simulink model "LRMate200Experimentor_RobotState"  (R2015b)
settings: Solver=FixedStepDiscrete  StartTime=0.0  StopTime=10.0  FixedStep=si.SolverTimeStep  RelTol=1e-3
model workspace (MATLAB code in the model file):
  | rsi = evalin('base', 'si.ri{1}');
undefined symbols (not defined in the file or in its folder): si
libraries: xpcethercatlib x171
(part 1 of 2)
settings Model: xpc_rtwmakecfg_data=_xpcethercatlib_  ParameterArgumentNames=rsi  Creator=rluser  LastModifiedBy=Chin
settings SolverCC: EnableConcurrentExecution=on
settings DataIOCC: SaveFormat=Array
settings OptimizationCC: BlockReduction=off  OptimizeBlockIOStorage=off  BufferReuse=off  GlobalBufferReuse=off  ExpressionFolding=off  LocalBlockOutputs=off
settings DebuggingCC: SolverPrmCheckMsg=warning
settings HardwareCC: ProdBitPerPointer=32  ProdLargestAtomicFloat=None  ProdWordSize=32  ProdLongLongMode=on  ProdHWDeviceType=Generic->32-bit x86 compatible
settings RTWCC: SystemTargetFile=slrt.tlc  TemplateMakefile=slrt_default_tmf  Description=Simulink Real-Time  RTWCompilerOptimization=on
settings CodeAppCC: MaxIdLength=120
settings SimulinkRealTimeCC: GeneratePreprocessorConditionals=Disable all
settings ConfigComp: CovModelRefEnable=Off  CovSFcnEnable=off

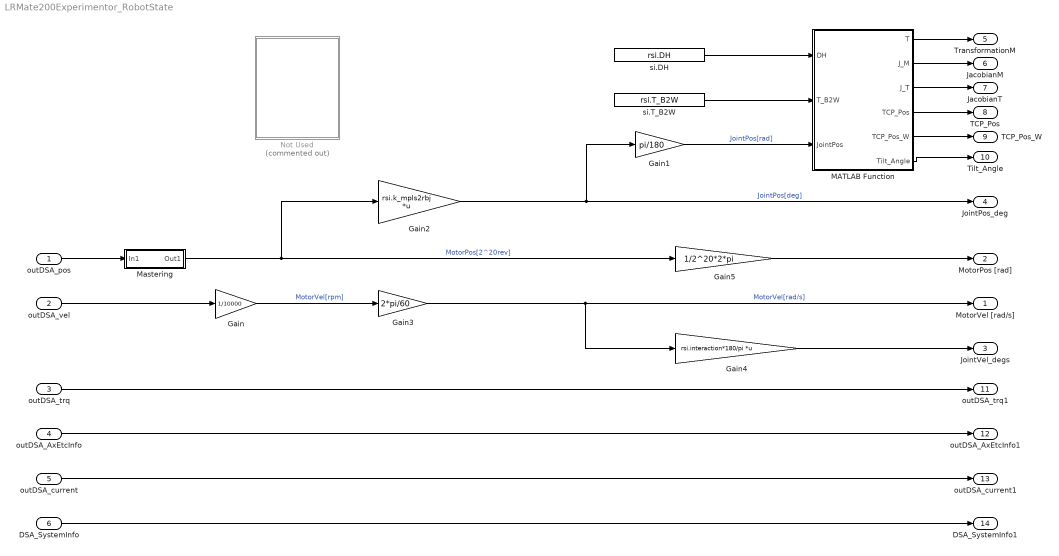
== system LRMate200Experimentor_RobotState ==
  outDSA_pos : Inport  PortDimensions=6
  outDSA_vel : Inport  Port=2  PortDimensions=6
  outDSA_trq : Inport  Port=3  PortDimensions=6
  outDSA_AxEtcInfo : Inport  Port=4  OutDataTypeStr=uint16  PortDimensions=6
  outDSA_current : Inport  Port=5  PortDimensions=6
  DSA_SystemInfo : Inport  Port=6  OutDataTypeStr=uint16
  Gain : Gain  Gain=1/10000  SampleTime=si.tsv
  Gain1 : Gain  Gain=pi/180
  Gain2 : Gain  Gain=rsi.k_mpls2rbj  Multiplication=Matrix(K*u)
  Gain3 : Gain  Gain=2*pi/60
  Gain4 : Gain  Gain=rsi.interaction*180/pi  Multiplication=Matrix(K*u)
  Gain5 : Gain  Gain=1/2^20*2*pi
  MATLAB Function : MATLAB Function  TreatAsAtomicUnit=on
  Mastering : Subsystem
  Not Used : Subsystem  Commented=on
  si.DH : Constant  Value=rsi.DH
  si.T_B2W : Constant  Value=rsi.T_B2W
  MotorVel [rad/s] : Outport
  MotorPos [rad] : Outport  Port=2
  JointVel_degs : Outport  Port=3
  JointPos_deg : Outport  Port=4
  TransformationM : Outport  Port=5
  JacobianM : Outport  Port=6
  JacobianT : Outport  Port=7
  TCP_Pos : Outport  Port=8
  TCP_Pos_W : Outport  Port=9
  Tilt_Angle : Outport  Port=10
  outDSA_trq1 : Outport  Port=11
  outDSA_AxEtcInfo1 : Outport  Port=12
  outDSA_current1 : Outport  Port=13
  DSA_SystemInfo1 : Outport  Port=14
  wires:
  DSA_SystemInfo/1 -> DSA_SystemInfo1/1
  outDSA_current/1 -> outDSA_current1/1
  outDSA_AxEtcInfo/1 -> outDSA_AxEtcInfo1/1
  outDSA_trq/1 -> outDSA_trq1/1
  outDSA_pos/1 -> Mastering/1(In1)
  Gain/1 -> Gain3/1  "MotorVel[rpm]"
  Gain2/1 -> JointPos_deg/1, Gain1/1  "JointPos[deg]"
  Gain3/1 -> MotorVel [rad/s]/1, Gain4/1  "MotorVel[rad/s]"
  si.DH/1 -> MATLAB Function/1(DH)
  MATLAB Function/1(T) -> TransformationM/1
  Gain4/1 -> JointVel_degs/1
  MATLAB Function/2(J_M) -> JacobianM/1
  Gain5/1 -> MotorPos [rad]/1
  Mastering/1(Out1) -> Gain5/1, Gain2/1  "MotorPos[2^20rev]"
  outDSA_vel/1 -> Gain/1
  MATLAB Function/3(J_T) -> JacobianT/1
  Gain1/1 -> MATLAB Function/3(JointPos)  "JointPos[rad]"
  MATLAB Function/4(TCP_Pos) -> TCP_Pos/1
  MATLAB Function/6(Tilt_Angle) -> Tilt_Angle/1
  si.T_B2W/1 -> MATLAB Function/2(T_B2W)
  MATLAB Function/5(TCP_Pos_W) -> TCP_Pos_W/1

== system LRMate200Experimentor_RobotState/Mastering ==
  note: モータ角度
      | [10^6*FlexFeedGear/rev]
  note: モータ角度[2^20/rev]
  note: モータ角度[2^20/rev]
  note: モータ角度[2^19/rev]
  In1 : Inport
  Add : Sum  Inputs=+-
  Gain : Gain  Gain=1./si.DSA_FlexFeedGear/1e6*2^20
  Gain1 : Gain  Gain=2
  MasterCount : Constant  Value=rsi.MasterCount  SampleTime=si.tsv
  Out1 : Outport
  wires:
  MasterCount/1 -> Gain1/1
  In1/1 -> Gain/1
  Add/1 -> Out1/1
  Gain/1 -> Add/1
  Gain1/1 -> Add/2

== system LRMate200Experimentor_RobotState/Not Used ==
  DSA SYSTEM : Subsystem  Commented=on
      settings: MinAlgLoopOccurrences=on
  DSA System Variant : Subsystem  Commented=on  Variant=on
  MATLAB Function : MATLAB Function  TreatAsAtomicUnit=on
  MATLAB Function1 : MATLAB Function  Commented=on  TreatAsAtomicUnit=on

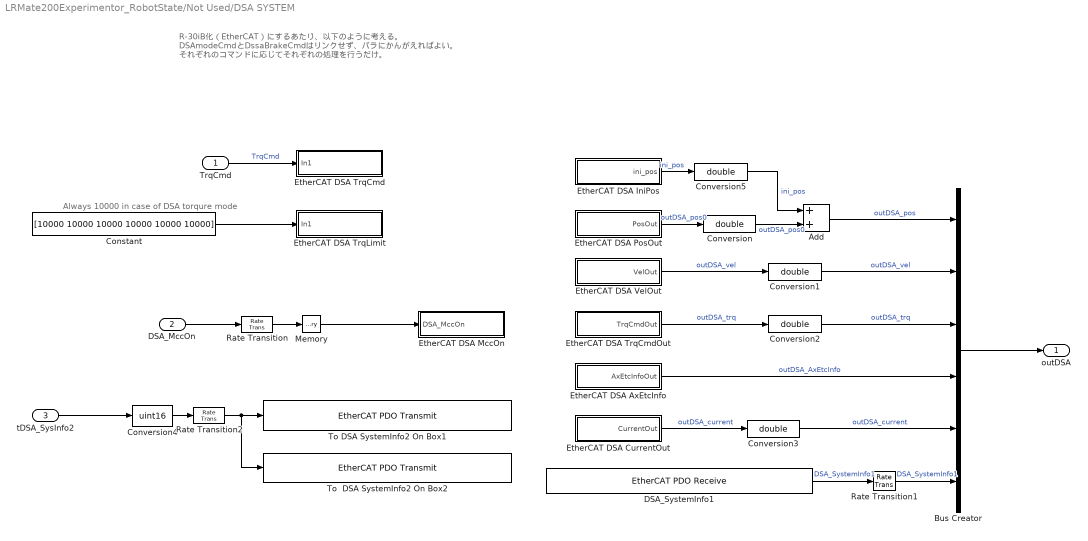
== system LRMate200Experimentor_RobotState/Not Used/DSA SYSTEM ==
  note: Always 10000 in case of DSA torqure mode
  note: R-30iB化（EtherCAT）にするあたり、以下のように考える。
      |
      | DSAmodeCmdとDssaBrakeCmdはリンクせず、パラにかんがえればよい。
      | それぞれのコマンドに応じてそれぞれの処理を行うだけ。
  TrqCmd : Inport
  DSA_MccOn : Inport  Port=2
  tDSA_SysInfo2 : Inport  Port=3
  Add : Sum
  Bus Creator : BusCreator  Inputs=6
  Constant : Constant  Value=[10000 10000 10000 10000 10000 10000]  SampleTime=si.etsv
  Conversion{,1..3,5} (5 alike) : DataTypeConversion  OutDataTypeStr=double
  Conversion4 : DataTypeConversion  OutDataTypeStr=uint16
  DSA_SystemInfo1 : xpcethercatlib/EtherCAT PDO Receive  Priority=2  sig_name=Box 1 (Degital Servo Adapter).NS-IN-SYS-DCIF.NSIS01  sig_offset=1352  sig_type=uint16  type_size=16  sig_dim=1  device_id=0  sample_time=0.000250
  EtherCAT DSA AxEtcInfo : Subsystem
  EtherCAT DSA CurrentOut : Subsystem
  EtherCAT DSA IniPos : Subsystem
  EtherCAT DSA MccOn : Subsystem
  EtherCAT DSA PosOut : Subsystem
  EtherCAT DSA TrqCmd : Subsystem
  EtherCAT DSA TrqCmdOut : Subsystem
  EtherCAT DSA TrqLimit : Subsystem
  EtherCAT DSA VelOut : Subsystem
  Memory : Memory
  Rate Transition : RateTransition
  Rate Transition1 : RateTransition  OutPortSampleTime=si.tsv
  Rate Transition2 : RateTransition
  To  DSA SystemInfo2 On Box2 : xpcethercatlib/EtherCAT PDO Transmit   Priority=3  sig_name=Box 2 (Degital Servo Adapter).NS-OUT-SYS-DCIF.NSOS01  sig_offset=3656  sig_type=uint16  type_size=16  sig_dim=1  device_id=0  sample_time=0.000250
  To DSA SystemInfo2 On Box1 : xpcethercatlib/EtherCAT PDO Transmit   Priority=3  sig_name=Box 1 (Degital Servo Adapter).NS-OUT-SYS-DCIF.NSOS01  sig_offset=1352  sig_type=uint16  type_size=16  sig_dim=1  device_id=0  sample_time=0.000250
  outDSA : Outport
  wires:
  EtherCAT DSA VelOut/1(VelOut) -> Conversion1/1  "outDSA_vel"
  EtherCAT DSA PosOut/1(PosOut) -> Conversion/1  "outDSA_pos0"
  EtherCAT DSA TrqCmdOut/1(TrqCmdOut) -> Conversion2/1  "outDSA_trq"
  EtherCAT DSA AxEtcInfo/1(AxEtcInfoOut) -> Bus Creator/4  "outDSA_AxEtcInfo"
  Bus Creator/1 -> outDSA/1
  TrqCmd/1 -> EtherCAT DSA TrqCmd/1(In1)  "TrqCmd"
  Conversion/1 -> Add/2  "outDSA_pos0"
  Conversion1/1 -> Bus Creator/2  "outDSA_vel"
  Conversion2/1 -> Bus Creator/3  "outDSA_trq"
  Memory/1 -> EtherCAT DSA MccOn/1(DSA_MccOn)
  Rate Transition/1 -> Memory/1
  EtherCAT DSA CurrentOut/1(CurrentOut) -> Conversion3/1  "outDSA_current"
  Conversion3/1 -> Bus Creator/5  "outDSA_current"
  DSA_MccOn/1 -> Rate Transition/1
  Rate Transition2/1 -> To  DSA SystemInfo2 On Box2/1, To DSA SystemInfo2 On Box1/1
  Conversion4/1 -> Rate Transition2/1
  tDSA_SysInfo2/1 -> Conversion4/1
  EtherCAT DSA IniPos/1(ini_pos) -> Conversion5/1  "ini_pos"
  Conversion5/1 -> Add/1  "ini_pos"
  Add/1 -> Bus Creator/1  "outDSA_pos"
  DSA_SystemInfo1/1 -> Rate Transition1/1  "DSA_SystemInfo1"
  Constant/1 -> EtherCAT DSA TrqLimit/1(In1)
  Rate Transition1/1 -> Bus Creator/6  "DSA_SystemInfo1"

== system LRMate200Experimentor_RobotState/Not Used/DSA System Variant ==
  note: 1) Add Subsystem or Model blocks as valid variant choices.
      | 2) You cannot connect blocks at this level. At simulation, connectivity is automatically
      | determined, based on the active variant and port name matching.
  MotorTrqCmd[DSA] : Inport
  DSA_MccOn : Inport  Port=2
  tDSA_SysInfo2 : Inport  Port=3
  DSA System (Robot 1) : Subsystem  VariantControl=robot_no == 1
      settings: MinAlgLoopOccurrences=on
  DSA System (Robot 2) : Subsystem  TreatAsAtomicUnit=on  VariantControl=robot_no == 2
      settings: MinAlgLoopOccurrences=on
  Empty : Subsystem  VariantControl=robot_no == 0
  outDSA : Outport

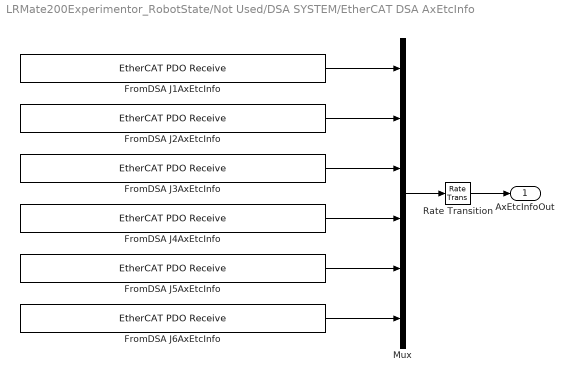
== system LRMate200Experimentor_RobotState/Not Used/DSA SYSTEM/EtherCAT DSA AxEtcInfo ==
  FromDSA J1AxEtcInfo : xpcethercatlib/EtherCAT PDO Receive  Priority=2  sig_name=Box 1 (Degital Servo Adapter).NS-IN-AX01.AX01-NSI07  sig_offset=1704  sig_type=uint16  type_size=16  sig_dim=1  device_id=0  sample_time=0.000250
  FromDSA J2AxEtcInfo : xpcethercatlib/EtherCAT PDO Receive  Priority=2  sig_name=Box 1 (Degital Servo Adapter).NS-IN-AX02.AX02-NSI07  sig_offset=1896  sig_type=uint16  type_size=16  sig_dim=1  device_id=0  sample_time=0.000250
  FromDSA J3AxEtcInfo : xpcethercatlib/EtherCAT PDO Receive  Priority=2  sig_name=Box 1 (Degital Servo Adapter).NS-IN-AX03.AX03-NSI07  sig_offset=2088  sig_type=uint16  type_size=16  sig_dim=1  device_id=0  sample_time=0.000250
  FromDSA J4AxEtcInfo : xpcethercatlib/EtherCAT PDO Receive  Priority=2  sig_name=Box 1 (Degital Servo Adapter).NS-IN-AX04.AX04-NSI07  sig_offset=2280  sig_type=uint16  type_size=16  sig_dim=1  device_id=0  sample_time=0.000250
  FromDSA J5AxEtcInfo : xpcethercatlib/EtherCAT PDO Receive  Priority=2  sig_name=Box 2 (Degital Servo Adapter).NS-IN-AX01.AX01-NSI07  sig_offset=4008  sig_type=uint16  type_size=16  sig_dim=1  device_id=0  sample_time=0.000250
  FromDSA J6AxEtcInfo : xpcethercatlib/EtherCAT PDO Receive  Priority=2  sig_name=Box 2 (Degital Servo Adapter).NS-IN-AX02.AX02-NSI07  sig_offset=4200  sig_type=uint16  type_size=16  sig_dim=1  device_id=0  sample_time=0.000250
  Mux : Mux  Inputs=6
  Rate Transition : RateTransition  OutPortSampleTime=si.tsv
  AxEtcInfoOut : Outport
  wires:
  FromDSA J6AxEtcInfo/1 -> Mux/6
  FromDSA J4AxEtcInfo/1 -> Mux/4
  FromDSA J2AxEtcInfo/1 -> Mux/2
  FromDSA J5AxEtcInfo/1 -> Mux/5
  FromDSA J3AxEtcInfo/1 -> Mux/3
  FromDSA J1AxEtcInfo/1 -> Mux/1
  Mux/1 -> Rate Transition/1
  Rate Transition/1 -> AxEtcInfoOut/1

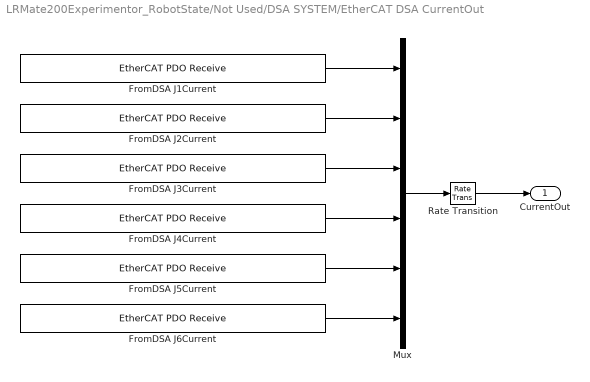
== system LRMate200Experimentor_RobotState/Not Used/DSA SYSTEM/EtherCAT DSA CurrentOut ==
  FromDSA J1Current : xpcethercatlib/EtherCAT PDO Receive  Priority=2  sig_name=Box 1 (Degital Servo Adapter).HS-IN-AX01.AX01-HSI03  sig_offset=360  sig_type=int16  type_size=16  sig_dim=1  device_id=0  sample_time=0.000250
  FromDSA J2Current : xpcethercatlib/EtherCAT PDO Receive  Priority=2  sig_name=Box 1 (Degital Servo Adapter).HS-IN-AX02.AX02-HSI03  sig_offset=616  sig_type=int16  type_size=16  sig_dim=1  device_id=0  sample_time=0.000250
  FromDSA J3Current : xpcethercatlib/EtherCAT PDO Receive  Priority=2  sig_name=Box 1 (Degital Servo Adapter).HS-IN-AX03.AX03-HSI03  sig_offset=872  sig_type=int16  type_size=16  sig_dim=1  device_id=0  sample_time=0.000250
  FromDSA J4Current : xpcethercatlib/EtherCAT PDO Receive  Priority=2  sig_name=Box 1 (Degital Servo Adapter).HS-IN-AX04.AX04-HSI03  sig_offset=1128  sig_type=int16  type_size=16  sig_dim=1  device_id=0  sample_time=0.000250
  FromDSA J5Current : xpcethercatlib/EtherCAT PDO Receive  Priority=2  sig_name=Box 2 (Degital Servo Adapter).HS-IN-AX01.AX01-HSI03  sig_offset=2664  sig_type=int16  type_size=16  sig_dim=1  device_id=0  sample_time=0.000250
  FromDSA J6Current : xpcethercatlib/EtherCAT PDO Receive  Priority=2  sig_name=Box 2 (Degital Servo Adapter).HS-IN-AX02.AX02-HSI03  sig_offset=2920  sig_type=int16  type_size=16  sig_dim=1  device_id=0  sample_time=0.000250
  Mux : Mux  Inputs=6
  Rate Transition : RateTransition  OutPortSampleTime=si.tsv
  CurrentOut : Outport
  wires:
  FromDSA J6Current/1 -> Mux/6
  FromDSA J4Current/1 -> Mux/4
  FromDSA J2Current/1 -> Mux/2
  FromDSA J5Current/1 -> Mux/5
  FromDSA J3Current/1 -> Mux/3
  FromDSA J1Current/1 -> Mux/1
  Mux/1 -> Rate Transition/1
  Rate Transition/1 -> CurrentOut/1

== system LRMate200Experimentor_RobotState/Not Used/DSA SYSTEM/EtherCAT DSA IniPos ==
  FromDSA J1IniPos : xpcethercatlib/EtherCAT PDO Receive  Priority=2  sig_name=Box 1 (Degital Servo Adapter).NS-IN-AX01.AX01-NSI02  sig_offset=1624  sig_type=int32  type_size=32  sig_dim=1  device_id=0  sample_time=0.000250
  FromDSA J2IniPos : xpcethercatlib/EtherCAT PDO Receive  Priority=2  sig_name=Box 1 (Degital Servo Adapter).NS-IN-AX02.AX02-NSI02  sig_offset=1816  sig_type=int32  type_size=32  sig_dim=1  device_id=0  sample_time=0.000250
  FromDSA J3IniPos : xpcethercatlib/EtherCAT PDO Receive  Priority=2  sig_name=Box 1 (Degital Servo Adapter).NS-IN-AX03.AX03-NSI02  sig_offset=2008  sig_type=int32  type_size=32  sig_dim=1  device_id=0  sample_time=0.000250
  FromDSA J4IniPos : xpcethercatlib/EtherCAT PDO Receive  Priority=2  sig_name=Box 1 (Degital Servo Adapter).NS-IN-AX04.AX04-NSI02  sig_offset=2200  sig_type=int32  type_size=32  sig_dim=1  device_id=0  sample_time=0.000250
  FromDSA J5IniPos : xpcethercatlib/EtherCAT PDO Receive  Priority=2  sig_name=Box 2 (Degital Servo Adapter).NS-IN-AX01.AX01-NSI02  sig_offset=3928  sig_type=int32  type_size=32  sig_dim=1  device_id=0  sample_time=0.000250
  FromDSA J6IniPos : xpcethercatlib/EtherCAT PDO Receive  Priority=2  sig_name=Box 2 (Degital Servo Adapter).NS-IN-AX02.AX02-NSI02  sig_offset=4120  sig_type=int32  type_size=32  sig_dim=1  device_id=0  sample_time=0.000250
  Mux : Mux  Inputs=6
  Rate Transition : RateTransition  OutPortSampleTime=si.tsv
  ini_pos : Outport
  wires:
  FromDSA J6IniPos/1 -> Mux/6
  FromDSA J4IniPos/1 -> Mux/4
  FromDSA J2IniPos/1 -> Mux/2
  FromDSA J5IniPos/1 -> Mux/5
  FromDSA J3IniPos/1 -> Mux/3
  FromDSA J1IniPos/1 -> Mux/1
  Mux/1 -> Rate Transition/1
  Rate Transition/1 -> ini_pos/1

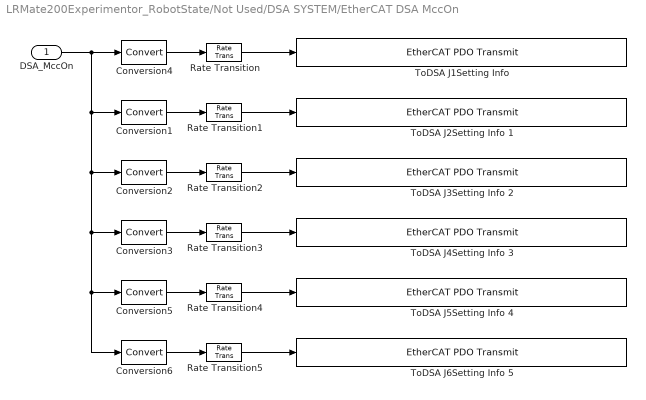
== system LRMate200Experimentor_RobotState/Not Used/DSA SYSTEM/EtherCAT DSA MccOn ==
  DSA_MccOn : Inport
  Conversion{1..6} (6 alike) : DataTypeConversion
  Rate Transition{,1..5} (6 alike) : RateTransition
  "ToDSA J1Setting Info " : xpcethercatlib/EtherCAT PDO Transmit   Priority=3  sig_name=Box 1 (Degital Servo Adapter).NS-OUT-AX01.AX01-NSO03  sig_offset=1640  sig_type=uint16  type_size=16  sig_dim=1  device_id=0  sample_time=0.000250
  ToDSA J2Setting Info 1 : xpcethercatlib/EtherCAT PDO Transmit   Priority=3  sig_name=Box 1 (Degital Servo Adapter).NS-OUT-AX02.AX02-NSO03  sig_offset=1896  sig_type=uint16  type_size=16  sig_dim=1  device_id=0  sample_time=0.000250
  ToDSA J3Setting Info 2 : xpcethercatlib/EtherCAT PDO Transmit   Priority=3  sig_name=Box 1 (Degital Servo Adapter).NS-OUT-AX03.AX03-NSO03  sig_offset=2152  sig_type=uint16  type_size=16  sig_dim=1  device_id=0  sample_time=0.000250
  ToDSA J4Setting Info 3 : xpcethercatlib/EtherCAT PDO Transmit   Priority=3  sig_name=Box 1 (Degital Servo Adapter).NS-OUT-AX04.AX04-NSO03  sig_offset=2408  sig_type=uint16  type_size=16  sig_dim=1  device_id=0  sample_time=0.000250
  ToDSA J5Setting Info 4 : xpcethercatlib/EtherCAT PDO Transmit   Priority=3  sig_name=Box 2 (Degital Servo Adapter).NS-OUT-AX01.AX01-NSO03  sig_offset=3944  sig_type=uint16  type_size=16  sig_dim=1  device_id=0  sample_time=0.000250
  ToDSA J6Setting Info 5 : xpcethercatlib/EtherCAT PDO Transmit   Priority=3  sig_name=Box 2 (Degital Servo Adapter).NS-OUT-AX02.AX02-NSO03  sig_offset=4200  sig_type=uint16  type_size=16  sig_dim=1  device_id=0  sample_time=0.000250
  wires:
  Rate Transition/1 -> "ToDSA J1Setting Info "/1
  Conversion4/1 -> Rate Transition/1
  DSA_MccOn/1 -> Conversion6/1, Conversion5/1, Conversion3/1, Conversion2/1, Conversion1/1, Conversion4/1
  Rate Transition1/1 -> ToDSA J2Setting Info 1/1
  Conversion1/1 -> Rate Transition1/1
  Rate Transition2/1 -> ToDSA J3Setting Info 2/1
  Conversion2/1 -> Rate Transition2/1
  Rate Transition3/1 -> ToDSA J4Setting Info 3/1
  Conversion3/1 -> Rate Transition3/1
  Rate Transition4/1 -> ToDSA J5Setting Info 4/1
  Conversion5/1 -> Rate Transition4/1
  Rate Transition5/1 -> ToDSA J6Setting Info 5/1
  Conversion6/1 -> Rate Transition5/1

== system LRMate200Experimentor_RobotState/Not Used/DSA SYSTEM/EtherCAT DSA PosOut ==
  FromDSA J1Pos : xpcethercatlib/EtherCAT PDO Receive  Priority=2  sig_name=Box 1 (Degital Servo Adapter).HS-IN-AX01.AX01-HSI12  sig_offset=504  sig_type=int32  type_size=32  sig_dim=1  device_id=0  sample_time=0.000250
  FromDSA J2Pos : xpcethercatlib/EtherCAT PDO Receive  Priority=2  sig_name=Box 1 (Degital Servo Adapter).HS-IN-AX02.AX02-HSI12  sig_offset=760  sig_type=int32  type_size=32  sig_dim=1  device_id=0  sample_time=0.000250
  FromDSA J3Pos : xpcethercatlib/EtherCAT PDO Receive  Priority=2  sig_name=Box 1 (Degital Servo Adapter).HS-IN-AX03.AX03-HSI12  sig_offset=1016  sig_type=int32  type_size=32  sig_dim=1  device_id=0  sample_time=0.000250
  FromDSA J4Pos : xpcethercatlib/EtherCAT PDO Receive  Priority=2  sig_name=Box 1 (Degital Servo Adapter).HS-IN-AX04.AX04-HSI12  sig_offset=1272  sig_type=int32  type_size=32  sig_dim=1  device_id=0  sample_time=0.000250
  FromDSA J5Pos : xpcethercatlib/EtherCAT PDO Receive  Priority=2  sig_name=Box 2 (Degital Servo Adapter).HS-IN-AX01.AX01-HSI12  sig_offset=2808  sig_type=int32  type_size=32  sig_dim=1  device_id=0  sample_time=0.000250
  FromDSA J6Pos : xpcethercatlib/EtherCAT PDO Receive  Priority=2  sig_name=Box 2 (Degital Servo Adapter).HS-IN-AX02.AX02-HSI12  sig_offset=3064  sig_type=int32  type_size=32  sig_dim=1  device_id=0  sample_time=0.000250
  Mux : Mux  Inputs=6
  Rate Transition : RateTransition  OutPortSampleTime=si.tsv
  PosOut : Outport
  wires:
  FromDSA J6Pos/1 -> Mux/6
  FromDSA J4Pos/1 -> Mux/4
  FromDSA J2Pos/1 -> Mux/2
  FromDSA J5Pos/1 -> Mux/5
  FromDSA J3Pos/1 -> Mux/3
  FromDSA J1Pos/1 -> Mux/1
  Mux/1 -> Rate Transition/1
  Rate Transition/1 -> PosOut/1

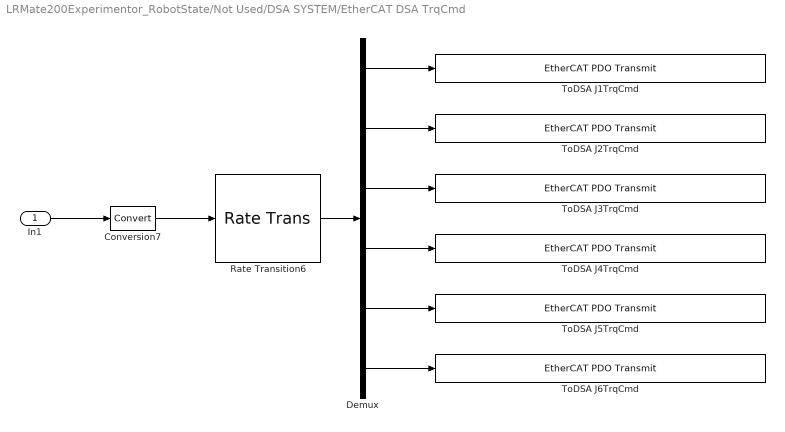
== system LRMate200Experimentor_RobotState/Not Used/DSA SYSTEM/EtherCAT DSA TrqCmd ==
  In1 : Inport
  Conversion7 : DataTypeConversion
  Demux : Demux  Outputs=6
  Rate Transition6 : RateTransition
  "ToDSA J1TrqCmd " : xpcethercatlib/EtherCAT PDO Transmit   Priority=3  sig_name=Box 1 (Degital Servo Adapter).HS-OUT-AX01.AX01-HSO04  sig_offset=376  sig_type=int16  type_size=16  sig_dim=1  device_id=0  sample_time=0.000250
  ToDSA J2TrqCmd : xpcethercatlib/EtherCAT PDO Transmit   Priority=3  sig_name=Box 1 (Degital Servo Adapter).HS-OUT-AX02.AX02-HSO04  sig_offset=632  sig_type=int16  type_size=16  sig_dim=1  device_id=0  sample_time=0.000250
  ToDSA J3TrqCmd : xpcethercatlib/EtherCAT PDO Transmit   Priority=3  sig_name=Box 1 (Degital Servo Adapter).HS-OUT-AX03.AX03-HSO04  sig_offset=888  sig_type=int16  type_size=16  sig_dim=1  device_id=0  sample_time=0.000250
  ToDSA J4TrqCmd : xpcethercatlib/EtherCAT PDO Transmit   Priority=3  sig_name=Box 1 (Degital Servo Adapter).HS-OUT-AX04.AX04-HSO04  sig_offset=1144  sig_type=int16  type_size=16  sig_dim=1  device_id=0  sample_time=0.000250
  ToDSA J5TrqCmd : xpcethercatlib/EtherCAT PDO Transmit   Priority=3  sig_name=Box 2 (Degital Servo Adapter).HS-OUT-AX01.AX01-HSO04  sig_offset=2680  sig_type=int16  type_size=16  sig_dim=1  device_id=0  sample_time=0.000250
  ToDSA J6TrqCmd : xpcethercatlib/EtherCAT PDO Transmit   Priority=3  sig_name=Box 2 (Degital Servo Adapter).HS-OUT-AX02.AX02-HSO04  sig_offset=2936  sig_type=int16  type_size=16  sig_dim=1  device_id=0  sample_time=0.000250
  wires:
  In1/1 -> Conversion7/1
  Conversion7/1 -> Rate Transition6/1
  Rate Transition6/1 -> Demux/1
  Demux/1 -> "ToDSA J1TrqCmd "/1
  Demux/2 -> ToDSA J2TrqCmd/1
  Demux/3 -> ToDSA J3TrqCmd/1
  Demux/4 -> ToDSA J4TrqCmd/1
  Demux/5 -> ToDSA J5TrqCmd/1
  Demux/6 -> ToDSA J6TrqCmd/1

== system LRMate200Experimentor_RobotState/Not Used/DSA SYSTEM/EtherCAT DSA TrqCmdOut ==
  FromDSA J1TrqCmd : xpcethercatlib/EtherCAT PDO Receive  Priority=2  sig_name=Box 1 (Degital Servo Adapter).HS-IN-AX01.AX01-HSI02  sig_offset=344  sig_type=int16  type_size=16  sig_dim=1  device_id=0  sample_time=0.000250
  FromDSA J2TrqCmd : xpcethercatlib/EtherCAT PDO Receive  Priority=2  sig_name=Box 1 (Degital Servo Adapter).HS-IN-AX02.AX02-HSI02  sig_offset=600  sig_type=int16  type_size=16  sig_dim=1  device_id=0  sample_time=0.000250
  FromDSA J3TrqCmd2 : xpcethercatlib/EtherCAT PDO Receive  Priority=2  sig_name=Box 1 (Degital Servo Adapter).HS-IN-AX03.AX03-HSI02  sig_offset=856  sig_type=int16  type_size=16  sig_dim=1  device_id=0  sample_time=0.000250
  FromDSA J4TrqCmd3 : xpcethercatlib/EtherCAT PDO Receive  Priority=2  sig_name=Box 1 (Degital Servo Adapter).HS-IN-AX04.AX04-HSI02  sig_offset=1112  sig_type=int16  type_size=16  sig_dim=1  device_id=0  sample_time=0.000250
  FromDSA J5TrqCmd4 : xpcethercatlib/EtherCAT PDO Receive  Priority=2  sig_name=Box 2 (Degital Servo Adapter).HS-IN-AX01.AX01-HSI02  sig_offset=2648  sig_type=int16  type_size=16  sig_dim=1  device_id=0  sample_time=0.000250
  FromDSA J6TrqCmd5 : xpcethercatlib/EtherCAT PDO Receive  Priority=2  sig_name=Box 2 (Degital Servo Adapter).HS-IN-AX02.AX02-HSI02  sig_offset=2904  sig_type=int16  type_size=16  sig_dim=1  device_id=0  sample_time=0.000250
  Mux : Mux  Inputs=6
  Rate Transition : RateTransition  OutPortSampleTime=si.tsv
  TrqCmdOut : Outport
  wires:
  FromDSA J6TrqCmd5/1 -> Mux/6
  FromDSA J4TrqCmd3/1 -> Mux/4
  FromDSA J2TrqCmd/1 -> Mux/2
  FromDSA J5TrqCmd4/1 -> Mux/5
  FromDSA J3TrqCmd2/1 -> Mux/3
  FromDSA J1TrqCmd/1 -> Mux/1
  Mux/1 -> Rate Transition/1
  Rate Transition/1 -> TrqCmdOut/1

== system LRMate200Experimentor_RobotState/Not Used/DSA SYSTEM/EtherCAT DSA TrqLimit ==
  In1 : Inport
  Conversion7 : DataTypeConversion
  Demux : Demux  Outputs=6
  "ToDSA J1TrqLimit " : xpcethercatlib/EtherCAT PDO Transmit   Priority=3  sig_name=Box 1 (Degital Servo Adapter).HS-OUT-AX01.AX01-HSO05  sig_offset=392  sig_type=int16  type_size=16  sig_dim=1  device_id=0  sample_time=0.000250
  ToDSA J2TrqLimit : xpcethercatlib/EtherCAT PDO Transmit   Priority=3  sig_name=Box 1 (Degital Servo Adapter).HS-OUT-AX02.AX02-HSO05  sig_offset=648  sig_type=int16  type_size=16  sig_dim=1  device_id=0  sample_time=0.000250
  ToDSA J3TrqLimit : xpcethercatlib/EtherCAT PDO Transmit   Priority=3  sig_name=Box 1 (Degital Servo Adapter).HS-OUT-AX03.AX03-HSO05  sig_offset=904  sig_type=int16  type_size=16  sig_dim=1  device_id=0  sample_time=0.000250
  ToDSA J4TrqLimit : xpcethercatlib/EtherCAT PDO Transmit   Priority=3  sig_name=Box 1 (Degital Servo Adapter).HS-OUT-AX04.AX04-HSO05  sig_offset=1160  sig_type=int16  type_size=16  sig_dim=1  device_id=0  sample_time=0.000250
  ToDSA J5TrqLimit : xpcethercatlib/EtherCAT PDO Transmit   Priority=3  sig_name=Box 2 (Degital Servo Adapter).HS-OUT-AX01.AX01-HSO05  sig_offset=2696  sig_type=int16  type_size=16  sig_dim=1  device_id=0  sample_time=0.000250
  ToDSA J6TrqLimit : xpcethercatlib/EtherCAT PDO Transmit   Priority=3  sig_name=Box 2 (Degital Servo Adapter).HS-OUT-AX02.AX02-HSO05  sig_offset=2952  sig_type=int16  type_size=16  sig_dim=1  device_id=0  sample_time=0.000250
  wires:
  In1/1 -> Conversion7/1
  Demux/1 -> "ToDSA J1TrqLimit "/1
  Demux/2 -> ToDSA J2TrqLimit/1
  Demux/3 -> ToDSA J3TrqLimit/1
  Demux/4 -> ToDSA J4TrqLimit/1
  Demux/5 -> ToDSA J5TrqLimit/1
  Demux/6 -> ToDSA J6TrqLimit/1
  Conversion7/1 -> Demux/1

== system LRMate200Experimentor_RobotState/Not Used/DSA SYSTEM/EtherCAT DSA VelOut ==
  FromDSA J1Vel : xpcethercatlib/EtherCAT PDO Receive  Priority=2  sig_name=Box 1 (Degital Servo Adapter).HS-IN-AX01.AX01-HSI10  sig_offset=472  sig_type=int32  type_size=32  sig_dim=1  device_id=0  sample_time=0.000250
  FromDSA J2Vel : xpcethercatlib/EtherCAT PDO Receive  Priority=2  sig_name=Box 1 (Degital Servo Adapter).HS-IN-AX02.AX02-HSI10  sig_offset=728  sig_type=int32  type_size=32  sig_dim=1  device_id=0  sample_time=0.000250
  FromDSA J3Vel : xpcethercatlib/EtherCAT PDO Receive  Priority=2  sig_name=Box 1 (Degital Servo Adapter).HS-IN-AX03.AX03-HSI10  sig_offset=984  sig_type=int32  type_size=32  sig_dim=1  device_id=0  sample_time=0.000250
  FromDSA J4Vel : xpcethercatlib/EtherCAT PDO Receive  Priority=2  sig_name=Box 1 (Degital Servo Adapter).HS-IN-AX04.AX04-HSI10  sig_offset=1240  sig_type=int32  type_size=32  sig_dim=1  device_id=0  sample_time=0.000250
  FromDSA J5Vel : xpcethercatlib/EtherCAT PDO Receive  Priority=2  sig_name=Box 2 (Degital Servo Adapter).HS-IN-AX01.AX01-HSI10  sig_offset=2776  sig_type=int32  type_size=32  sig_dim=1  device_id=0  sample_time=0.000250
  FromDSA J6Vel : xpcethercatlib/EtherCAT PDO Receive  Priority=2  sig_name=Box 2 (Degital Servo Adapter).HS-IN-AX02.AX02-HSI10  sig_offset=3032  sig_type=int32  type_size=32  sig_dim=1  device_id=0  sample_time=0.000250
  Mux : Mux  Inputs=6
  Rate Transition : RateTransition  OutPortSampleTime=si.tsv
  VelOut : Outport
  wires:
  FromDSA J6Vel/1 -> Mux/6
  FromDSA J4Vel/1 -> Mux/4
  FromDSA J2Vel/1 -> Mux/2
  FromDSA J5Vel/1 -> Mux/5
  FromDSA J3Vel/1 -> Mux/3
  FromDSA J1Vel/1 -> Mux/1
  Rate Transition/1 -> VelOut/1
  Mux/1 -> Rate Transition/1

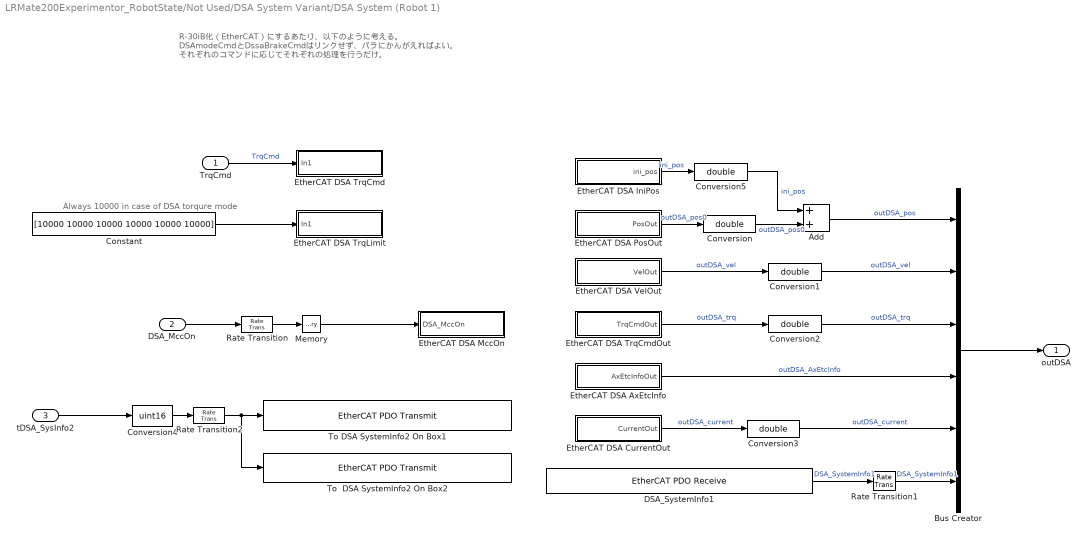
== system LRMate200Experimentor_RobotState/Not Used/DSA System Variant/DSA System (Robot 1) ==
  note: Always 10000 in case of DSA torqure mode
  note: R-30iB化（EtherCAT）にするあたり、以下のように考える。
      |
      | DSAmodeCmdとDssaBrakeCmdはリンクせず、パラにかんがえればよい。
      | それぞれのコマンドに応じてそれぞれの処理を行うだけ。
  TrqCmd : Inport
  DSA_MccOn : Inport  Port=2
  tDSA_SysInfo2 : Inport  Port=3
  Add : Sum
  Bus Creator : BusCreator  Inputs=6
  Constant : Constant  Value=[10000 10000 10000 10000 10000 10000]  SampleTime=si.etsv
  Conversion{,1..3,5} (5 alike) : DataTypeConversion  OutDataTypeStr=double
  Conversion4 : DataTypeConversion  OutDataTypeStr=uint16
  DSA_SystemInfo1 : xpcethercatlib/EtherCAT PDO Receive  Priority=2  sig_name=Box 1 (Degital Servo Adapter).NS-IN-SYS-DCIF.NSIS01  sig_offset=1352  sig_type=uint16  type_size=16  sig_dim=1  device_id=0  sample_time=0.000250
  EtherCAT DSA AxEtcInfo : Subsystem
  EtherCAT DSA CurrentOut : Subsystem
  EtherCAT DSA IniPos : Subsystem
  EtherCAT DSA MccOn : Subsystem
  EtherCAT DSA PosOut : Subsystem
  EtherCAT DSA TrqCmd : Subsystem
  EtherCAT DSA TrqCmdOut : Subsystem
  EtherCAT DSA TrqLimit : Subsystem
  EtherCAT DSA VelOut : Subsystem
  Memory : Memory
  Rate Transition : RateTransition
  Rate Transition1 : RateTransition  OutPortSampleTime=si.tsv
  Rate Transition2 : RateTransition
  To  DSA SystemInfo2 On Box2 : xpcethercatlib/EtherCAT PDO Transmit   Priority=3  sig_name=Box 2 (Degital Servo Adapter).NS-OUT-SYS-DCIF.NSOS01  sig_offset=3656  sig_type=uint16  type_size=16  sig_dim=1  device_id=0  sample_time=0.000250
  To DSA SystemInfo2 On Box1 : xpcethercatlib/EtherCAT PDO Transmit   Priority=3  sig_name=Box 1 (Degital Servo Adapter).NS-OUT-SYS-DCIF.NSOS01  sig_offset=1352  sig_type=uint16  type_size=16  sig_dim=1  device_id=0  sample_time=0.000250
  outDSA : Outport
  wires:
  EtherCAT DSA VelOut/1(VelOut) -> Conversion1/1  "outDSA_vel"
  EtherCAT DSA PosOut/1(PosOut) -> Conversion/1  "outDSA_pos0"
  EtherCAT DSA TrqCmdOut/1(TrqCmdOut) -> Conversion2/1  "outDSA_trq"
  EtherCAT DSA AxEtcInfo/1(AxEtcInfoOut) -> Bus Creator/4  "outDSA_AxEtcInfo"
  Bus Creator/1 -> outDSA/1
  TrqCmd/1 -> EtherCAT DSA TrqCmd/1(In1)  "TrqCmd"
  Conversion/1 -> Add/2  "outDSA_pos0"
  Conversion1/1 -> Bus Creator/2  "outDSA_vel"
  Conversion2/1 -> Bus Creator/3  "outDSA_trq"
  Memory/1 -> EtherCAT DSA MccOn/1(DSA_MccOn)
  Rate Transition/1 -> Memory/1
  EtherCAT DSA CurrentOut/1(CurrentOut) -> Conversion3/1  "outDSA_current"
  Conversion3/1 -> Bus Creator/5  "outDSA_current"
  DSA_MccOn/1 -> Rate Transition/1
  Rate Transition2/1 -> To  DSA SystemInfo2 On Box2/1, To DSA SystemInfo2 On Box1/1
  Conversion4/1 -> Rate Transition2/1
  tDSA_SysInfo2/1 -> Conversion4/1
  EtherCAT DSA IniPos/1(ini_pos) -> Conversion5/1  "ini_pos"
  Conversion5/1 -> Add/1  "ini_pos"
  Add/1 -> Bus Creator/1  "outDSA_pos"
  DSA_SystemInfo1/1 -> Rate Transition1/1  "DSA_SystemInfo1"
  Constant/1 -> EtherCAT DSA TrqLimit/1(In1)
  Rate Transition1/1 -> Bus Creator/6  "DSA_SystemInfo1"

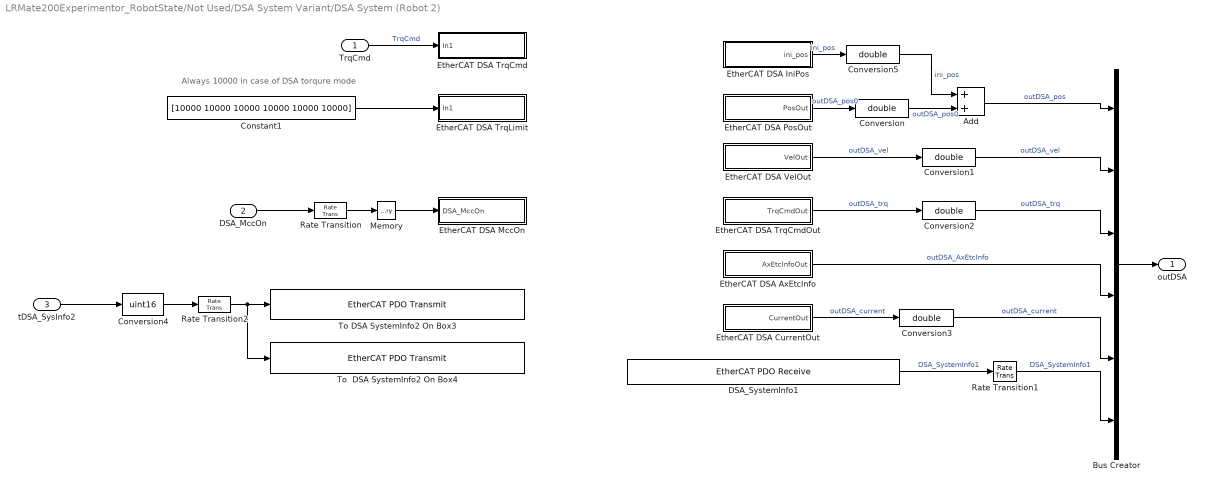
== system LRMate200Experimentor_RobotState/Not Used/DSA System Variant/DSA System (Robot 2) ==
  note: Always 10000 in case of DSA torqure mode
  TrqCmd : Inport
  DSA_MccOn : Inport  Port=2
  tDSA_SysInfo2 : Inport  Port=3
  Add : Sum
  Bus Creator : BusCreator  Inputs=6
  Constant1 : Constant  Value=[10000 10000 10000 10000 10000 10000]  SampleTime=si.etsv
  Conversion{,1..3,5} (5 alike) : DataTypeConversion  OutDataTypeStr=double
  Conversion4 : DataTypeConversion  OutDataTypeStr=uint16
  DSA_SystemInfo1 : xpcethercatlib/EtherCAT PDO Receive  Priority=2  sig_name=Box 3 (Degital Servo Adapter).NS-IN-SYS-DCIF.NSIS01  sig_offset=5960  sig_type=uint16  type_size=16  sig_dim=1  device_id=0  sample_time=0.000250
  EtherCAT DSA AxEtcInfo : Subsystem
  EtherCAT DSA CurrentOut : Subsystem
  EtherCAT DSA IniPos : Subsystem
  EtherCAT DSA MccOn : Subsystem
  EtherCAT DSA PosOut : Subsystem
  EtherCAT DSA TrqCmd : Subsystem
  EtherCAT DSA TrqCmdOut : Subsystem
  EtherCAT DSA TrqLimit : Subsystem
  EtherCAT DSA VelOut : Subsystem
  Memory : Memory
  Rate Transition : RateTransition
  Rate Transition1 : RateTransition  OutPortSampleTime=si.tsv
  Rate Transition2 : RateTransition
  To  DSA SystemInfo2 On Box4 : xpcethercatlib/EtherCAT PDO Transmit   Priority=3  sig_name=Box 4 (Degital Servo Adapter).NS-OUT-SYS-DCIF.NSOS01  sig_offset=8264  sig_type=uint16  type_size=16  sig_dim=1  device_id=0  sample_time=0.000250
  To DSA SystemInfo2 On Box3 : xpcethercatlib/EtherCAT PDO Transmit   Priority=3  sig_name=Box 3 (Degital Servo Adapter).NS-OUT-SYS-DCIF.NSOS01  sig_offset=5960  sig_type=uint16  type_size=16  sig_dim=1  device_id=0  sample_time=0.000250
  outDSA : Outport
  wires:
  EtherCAT DSA VelOut/1(VelOut) -> Conversion1/1  "outDSA_vel"
  EtherCAT DSA PosOut/1(PosOut) -> Conversion/1  "outDSA_pos0"
  EtherCAT DSA TrqCmdOut/1(TrqCmdOut) -> Conversion2/1  "outDSA_trq"
  EtherCAT DSA AxEtcInfo/1(AxEtcInfoOut) -> Bus Creator/4  "outDSA_AxEtcInfo"
  Bus Creator/1 -> outDSA/1
  TrqCmd/1 -> EtherCAT DSA TrqCmd/1(In1)  "TrqCmd"
  Conversion/1 -> Add/2  "outDSA_pos0"
  Conversion1/1 -> Bus Creator/2  "outDSA_vel"
  Conversion2/1 -> Bus Creator/3  "outDSA_trq"
  Memory/1 -> EtherCAT DSA MccOn/1(DSA_MccOn)
  Rate Transition/1 -> Memory/1
  EtherCAT DSA CurrentOut/1(CurrentOut) -> Conversion3/1  "outDSA_current"
  Conversion3/1 -> Bus Creator/5  "outDSA_current"
  DSA_MccOn/1 -> Rate Transition/1
  Rate Transition2/1 -> To  DSA SystemInfo2 On Box4/1, To DSA SystemInfo2 On Box3/1
  Conversion4/1 -> Rate Transition2/1
  tDSA_SysInfo2/1 -> Conversion4/1
  EtherCAT DSA IniPos/1(ini_pos) -> Conversion5/1  "ini_pos"
  Conversion5/1 -> Add/1  "ini_pos"
  Add/1 -> Bus Creator/1  "outDSA_pos"
  DSA_SystemInfo1/1 -> Rate Transition1/1  "DSA_SystemInfo1"
  Rate Transition1/1 -> Bus Creator/6  "DSA_SystemInfo1"
  Constant1/1 -> EtherCAT DSA TrqLimit/1(In1)

== system LRMate200Experimentor_RobotState/Not Used/DSA System Variant/Empty ==

== system LRMate200Experimentor_RobotState/Not Used/DSA System Variant/DSA System (Robot 1)/EtherCAT DSA AxEtcInfo ==
  FromDSA J1AxEtcInfo : xpcethercatlib/EtherCAT PDO Receive  Priority=2  sig_name=Box 1 (Degital Servo Adapter).NS-IN-AX01.AX01-NSI07  sig_offset=1704  sig_type=uint16  type_size=16  sig_dim=1  device_id=0  sample_time=0.000250
  FromDSA J2AxEtcInfo : xpcethercatlib/EtherCAT PDO Receive  Priority=2  sig_name=Box 1 (Degital Servo Adapter).NS-IN-AX02.AX02-NSI07  sig_offset=1896  sig_type=uint16  type_size=16  sig_dim=1  device_id=0  sample_time=0.000250
  FromDSA J3AxEtcInfo : xpcethercatlib/EtherCAT PDO Receive  Priority=2  sig_name=Box 1 (Degital Servo Adapter).NS-IN-AX03.AX03-NSI07  sig_offset=2088  sig_type=uint16  type_size=16  sig_dim=1  device_id=0  sample_time=0.000250
  FromDSA J4AxEtcInfo : xpcethercatlib/EtherCAT PDO Receive  Priority=2  sig_name=Box 1 (Degital Servo Adapter).NS-IN-AX04.AX04-NSI07  sig_offset=2280  sig_type=uint16  type_size=16  sig_dim=1  device_id=0  sample_time=0.000250
  FromDSA J5AxEtcInfo : xpcethercatlib/EtherCAT PDO Receive  Priority=2  sig_name=Box 2 (Degital Servo Adapter).NS-IN-AX01.AX01-NSI07  sig_offset=4008  sig_type=uint16  type_size=16  sig_dim=1  device_id=0  sample_time=0.000250
  FromDSA J6AxEtcInfo : xpcethercatlib/EtherCAT PDO Receive  Priority=2  sig_name=Box 2 (Degital Servo Adapter).NS-IN-AX02.AX02-NSI07  sig_offset=4200  sig_type=uint16  type_size=16  sig_dim=1  device_id=0  sample_time=0.000250
  Mux : Mux  Inputs=6
  Rate Transition : RateTransition  OutPortSampleTime=si.tsv
  AxEtcInfoOut : Outport
  wires:
  FromDSA J6AxEtcInfo/1 -> Mux/6
  FromDSA J4AxEtcInfo/1 -> Mux/4
  FromDSA J2AxEtcInfo/1 -> Mux/2
  FromDSA J5AxEtcInfo/1 -> Mux/5
  FromDSA J3AxEtcInfo/1 -> Mux/3
  FromDSA J1AxEtcInfo/1 -> Mux/1
  Mux/1 -> Rate Transition/1
  Rate Transition/1 -> AxEtcInfoOut/1

== system LRMate200Experimentor_RobotState/Not Used/DSA System Variant/DSA System (Robot 1)/EtherCAT DSA CurrentOut ==
  FromDSA J1Current : xpcethercatlib/EtherCAT PDO Receive  Priority=2  sig_name=Box 1 (Degital Servo Adapter).HS-IN-AX01.AX01-HSI03  sig_offset=360  sig_type=int16  type_size=16  sig_dim=1  device_id=0  sample_time=0.000250
  FromDSA J2Current : xpcethercatlib/EtherCAT PDO Receive  Priority=2  sig_name=Box 1 (Degital Servo Adapter).HS-IN-AX02.AX02-HSI03  sig_offset=616  sig_type=int16  type_size=16  sig_dim=1  device_id=0  sample_time=0.000250
  FromDSA J3Current : xpcethercatlib/EtherCAT PDO Receive  Priority=2  sig_name=Box 1 (Degital Servo Adapter).HS-IN-AX03.AX03-HSI03  sig_offset=872  sig_type=int16  type_size=16  sig_dim=1  device_id=0  sample_time=0.000250
  FromDSA J4Current : xpcethercatlib/EtherCAT PDO Receive  Priority=2  sig_name=Box 1 (Degital Servo Adapter).HS-IN-AX04.AX04-HSI03  sig_offset=1128  sig_type=int16  type_size=16  sig_dim=1  device_id=0  sample_time=0.000250
  FromDSA J5Current : xpcethercatlib/EtherCAT PDO Receive  Priority=2  sig_name=Box 2 (Degital Servo Adapter).HS-IN-AX01.AX01-HSI03  sig_offset=2664  sig_type=int16  type_size=16  sig_dim=1  device_id=0  sample_time=0.000250
  FromDSA J6Current : xpcethercatlib/EtherCAT PDO Receive  Priority=2  sig_name=Box 2 (Degital Servo Adapter).HS-IN-AX02.AX02-HSI03  sig_offset=2920  sig_type=int16  type_size=16  sig_dim=1  device_id=0  sample_time=0.000250
  Mux : Mux  Inputs=6
  Rate Transition : RateTransition  OutPortSampleTime=si.tsv
  CurrentOut : Outport
  wires:
  FromDSA J6Current/1 -> Mux/6
  FromDSA J4Current/1 -> Mux/4
  FromDSA J2Current/1 -> Mux/2
  FromDSA J5Current/1 -> Mux/5
  FromDSA J3Current/1 -> Mux/3
  FromDSA J1Current/1 -> Mux/1
  Mux/1 -> Rate Transition/1
  Rate Transition/1 -> CurrentOut/1

== system LRMate200Experimentor_RobotState/Not Used/DSA System Variant/DSA System (Robot 1)/EtherCAT DSA IniPos ==
  FromDSA J1IniPos : xpcethercatlib/EtherCAT PDO Receive  Priority=2  sig_name=Box 1 (Degital Servo Adapter).NS-IN-AX01.AX01-NSI02  sig_offset=1624  sig_type=int32  type_size=32  sig_dim=1  device_id=0  sample_time=0.000250
  FromDSA J2IniPos : xpcethercatlib/EtherCAT PDO Receive  Priority=2  sig_name=Box 1 (Degital Servo Adapter).NS-IN-AX02.AX02-NSI02  sig_offset=1816  sig_type=int32  type_size=32  sig_dim=1  device_id=0  sample_time=0.000250
  FromDSA J3IniPos : xpcethercatlib/EtherCAT PDO Receive  Priority=2  sig_name=Box 1 (Degital Servo Adapter).NS-IN-AX03.AX03-NSI02  sig_offset=2008  sig_type=int32  type_size=32  sig_dim=1  device_id=0  sample_time=0.000250
  FromDSA J4IniPos : xpcethercatlib/EtherCAT PDO Receive  Priority=2  sig_name=Box 1 (Degital Servo Adapter).NS-IN-AX04.AX04-NSI02  sig_offset=2200  sig_type=int32  type_size=32  sig_dim=1  device_id=0  sample_time=0.000250
  FromDSA J5IniPos : xpcethercatlib/EtherCAT PDO Receive  Priority=2  sig_name=Box 2 (Degital Servo Adapter).NS-IN-AX01.AX01-NSI02  sig_offset=3928  sig_type=int32  type_size=32  sig_dim=1  device_id=0  sample_time=0.000250
  FromDSA J6IniPos : xpcethercatlib/EtherCAT PDO Receive  Priority=2  sig_name=Box 2 (Degital Servo Adapter).NS-IN-AX02.AX02-NSI02  sig_offset=4120  sig_type=int32  type_size=32  sig_dim=1  device_id=0  sample_time=0.000250
  Mux : Mux  Inputs=6
  Rate Transition : RateTransition  OutPortSampleTime=si.tsv
  ini_pos : Outport
  wires:
  FromDSA J6IniPos/1 -> Mux/6
  FromDSA J4IniPos/1 -> Mux/4
  FromDSA J2IniPos/1 -> Mux/2
  FromDSA J5IniPos/1 -> Mux/5
  FromDSA J3IniPos/1 -> Mux/3
  FromDSA J1IniPos/1 -> Mux/1
  Mux/1 -> Rate Transition/1
  Rate Transition/1 -> ini_pos/1

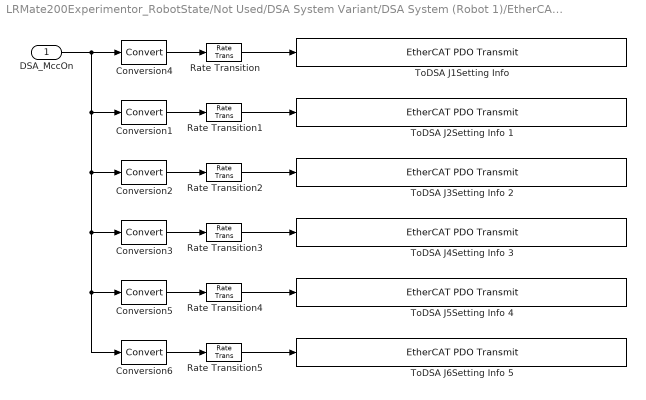
== system LRMate200Experimentor_RobotState/Not Used/DSA System Variant/DSA System (Robot 1)/EtherCAT DSA MccOn ==
  DSA_MccOn : Inport
  Conversion{1..6} (6 alike) : DataTypeConversion
  Rate Transition{,1..5} (6 alike) : RateTransition
  "ToDSA J1Setting Info " : xpcethercatlib/EtherCAT PDO Transmit   Priority=3  sig_name=Box 1 (Degital Servo Adapter).NS-OUT-AX01.AX01-NSO03  sig_offset=1640  sig_type=uint16  type_size=16  sig_dim=1  device_id=0  sample_time=0.000250
  ToDSA J2Setting Info 1 : xpcethercatlib/EtherCAT PDO Transmit   Priority=3  sig_name=Box 1 (Degital Servo Adapter).NS-OUT-AX02.AX02-NSO03  sig_offset=1896  sig_type=uint16  type_size=16  sig_dim=1  device_id=0  sample_time=0.000250
  ToDSA J3Setting Info 2 : xpcethercatlib/EtherCAT PDO Transmit   Priority=3  sig_name=Box 1 (Degital Servo Adapter).NS-OUT-AX03.AX03-NSO03  sig_offset=2152  sig_type=uint16  type_size=16  sig_dim=1  device_id=0  sample_time=0.000250
  ToDSA J4Setting Info 3 : xpcethercatlib/EtherCAT PDO Transmit   Priority=3  sig_name=Box 1 (Degital Servo Adapter).NS-OUT-AX04.AX04-NSO03  sig_offset=2408  sig_type=uint16  type_size=16  sig_dim=1  device_id=0  sample_time=0.000250
  ToDSA J5Setting Info 4 : xpcethercatlib/EtherCAT PDO Transmit   Priority=3  sig_name=Box 2 (Degital Servo Adapter).NS-OUT-AX01.AX01-NSO03  sig_offset=3944  sig_type=uint16  type_size=16  sig_dim=1  device_id=0  sample_time=0.000250
  ToDSA J6Setting Info 5 : xpcethercatlib/EtherCAT PDO Transmit   Priority=3  sig_name=Box 2 (Degital Servo Adapter).NS-OUT-AX02.AX02-NSO03  sig_offset=4200  sig_type=uint16  type_size=16  sig_dim=1  device_id=0  sample_time=0.000250
  wires:
  Rate Transition/1 -> "ToDSA J1Setting Info "/1
  Conversion4/1 -> Rate Transition/1
  DSA_MccOn/1 -> Conversion6/1, Conversion5/1, Conversion3/1, Conversion2/1, Conversion1/1, Conversion4/1
  Rate Transition1/1 -> ToDSA J2Setting Info 1/1
  Conversion1/1 -> Rate Transition1/1
  Rate Transition2/1 -> ToDSA J3Setting Info 2/1
  Conversion2/1 -> Rate Transition2/1
  Rate Transition3/1 -> ToDSA J4Setting Info 3/1
  Conversion3/1 -> Rate Transition3/1
  Rate Transition4/1 -> ToDSA J5Setting Info 4/1
  Conversion5/1 -> Rate Transition4/1
  Rate Transition5/1 -> ToDSA J6Setting Info 5/1
  Conversion6/1 -> Rate Transition5/1

== system LRMate200Experimentor_RobotState/Not Used/DSA System Variant/DSA System (Robot 1)/EtherCAT DSA PosOut ==
  FromDSA J1Pos : xpcethercatlib/EtherCAT PDO Receive  Priority=2  sig_name=Box 1 (Degital Servo Adapter).HS-IN-AX01.AX01-HSI12  sig_offset=504  sig_type=int32  type_size=32  sig_dim=1  device_id=0  sample_time=0.000250
  FromDSA J2Pos : xpcethercatlib/EtherCAT PDO Receive  Priority=2  sig_name=Box 1 (Degital Servo Adapter).HS-IN-AX02.AX02-HSI12  sig_offset=760  sig_type=int32  type_size=32  sig_dim=1  device_id=0  sample_time=0.000250
  FromDSA J3Pos : xpcethercatlib/EtherCAT PDO Receive  Priority=2  sig_name=Box 1 (Degital Servo Adapter).HS-IN-AX03.AX03-HSI12  sig_offset=1016  sig_type=int32  type_size=32  sig_dim=1  device_id=0  sample_time=0.000250
  FromDSA J4Pos : xpcethercatlib/EtherCAT PDO Receive  Priority=2  sig_name=Box 1 (Degital Servo Adapter).HS-IN-AX04.AX04-HSI12  sig_offset=1272  sig_type=int32  type_size=32  sig_dim=1  device_id=0  sample_time=0.000250
  FromDSA J5Pos : xpcethercatlib/EtherCAT PDO Receive  Priority=2  sig_name=Box 2 (Degital Servo Adapter).HS-IN-AX01.AX01-HSI12  sig_offset=2808  sig_type=int32  type_size=32  sig_dim=1  device_id=0  sample_time=0.000250
  FromDSA J6Pos : xpcethercatlib/EtherCAT PDO Receive  Priority=2  sig_name=Box 2 (Degital Servo Adapter).HS-IN-AX02.AX02-HSI12  sig_offset=3064  sig_type=int32  type_size=32  sig_dim=1  device_id=0  sample_time=0.000250
  Mux : Mux  Inputs=6
  Rate Transition : RateTransition  OutPortSampleTime=si.tsv
  PosOut : Outport
  wires:
  FromDSA J6Pos/1 -> Mux/6
  FromDSA J4Pos/1 -> Mux/4
  FromDSA J2Pos/1 -> Mux/2
  FromDSA J5Pos/1 -> Mux/5
  FromDSA J3Pos/1 -> Mux/3
  FromDSA J1Pos/1 -> Mux/1
  Mux/1 -> Rate Transition/1
  Rate Transition/1 -> PosOut/1

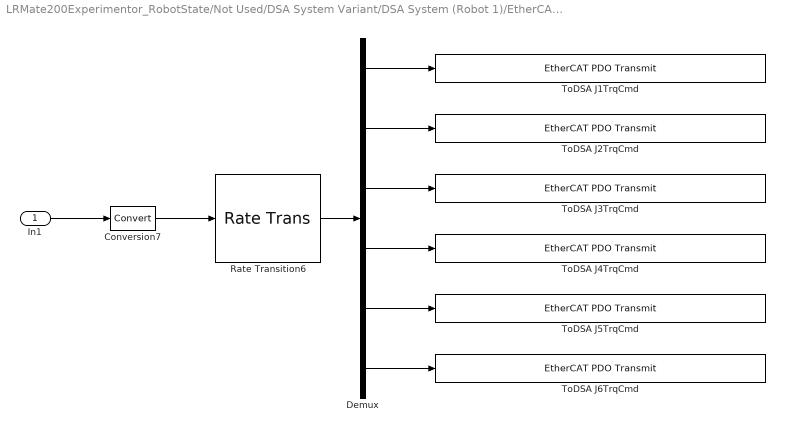
== system LRMate200Experimentor_RobotState/Not Used/DSA System Variant/DSA System (Robot 1)/EtherCAT DSA TrqCmd ==
  In1 : Inport
  Conversion7 : DataTypeConversion
  Demux : Demux  Outputs=6
  Rate Transition6 : RateTransition
  "ToDSA J1TrqCmd " : xpcethercatlib/EtherCAT PDO Transmit   Priority=3  sig_name=Box 1 (Degital Servo Adapter).HS-OUT-AX01.AX01-HSO04  sig_offset=376  sig_type=int16  type_size=16  sig_dim=1  device_id=0  sample_time=0.000250
  ToDSA J2TrqCmd : xpcethercatlib/EtherCAT PDO Transmit   Priority=3  sig_name=Box 1 (Degital Servo Adapter).HS-OUT-AX02.AX02-HSO04  sig_offset=632  sig_type=int16  type_size=16  sig_dim=1  device_id=0  sample_time=0.000250
  ToDSA J3TrqCmd : xpcethercatlib/EtherCAT PDO Transmit   Priority=3  sig_name=Box 1 (Degital Servo Adapter).HS-OUT-AX03.AX03-HSO04  sig_offset=888  sig_type=int16  type_size=16  sig_dim=1  device_id=0  sample_time=0.000250
  ToDSA J4TrqCmd : xpcethercatlib/EtherCAT PDO Transmit   Priority=3  sig_name=Box 1 (Degital Servo Adapter).HS-OUT-AX04.AX04-HSO04  sig_offset=1144  sig_type=int16  type_size=16  sig_dim=1  device_id=0  sample_time=0.000250
  ToDSA J5TrqCmd : xpcethercatlib/EtherCAT PDO Transmit   Priority=3  sig_name=Box 2 (Degital Servo Adapter).HS-OUT-AX01.AX01-HSO04  sig_offset=2680  sig_type=int16  type_size=16  sig_dim=1  device_id=0  sample_time=0.000250
  ToDSA J6TrqCmd : xpcethercatlib/EtherCAT PDO Transmit   Priority=3  sig_name=Box 2 (Degital Servo Adapter).HS-OUT-AX02.AX02-HSO04  sig_offset=2936  sig_type=int16  type_size=16  sig_dim=1  device_id=0  sample_time=0.000250
  wires:
  In1/1 -> Conversion7/1
  Conversion7/1 -> Rate Transition6/1
  Rate Transition6/1 -> Demux/1
  Demux/1 -> "ToDSA J1TrqCmd "/1
  Demux/2 -> ToDSA J2TrqCmd/1
  Demux/3 -> ToDSA J3TrqCmd/1
  Demux/4 -> ToDSA J4TrqCmd/1
  Demux/5 -> ToDSA J5TrqCmd/1
  Demux/6 -> ToDSA J6TrqCmd/1

== system LRMate200Experimentor_RobotState/Not Used/DSA System Variant/DSA System (Robot 1)/EtherCAT DSA TrqCmdOut ==
  FromDSA J1TrqCmd : xpcethercatlib/EtherCAT PDO Receive  Priority=2  sig_name=Box 1 (Degital Servo Adapter).HS-IN-AX01.AX01-HSI02  sig_offset=344  sig_type=int16  type_size=16  sig_dim=1  device_id=0  sample_time=0.000250
  FromDSA J2TrqCmd : xpcethercatlib/EtherCAT PDO Receive  Priority=2  sig_name=Box 1 (Degital Servo Adapter).HS-IN-AX02.AX02-HSI02  sig_offset=600  sig_type=int16  type_size=16  sig_dim=1  device_id=0  sample_time=0.000250
  FromDSA J3TrqCmd2 : xpcethercatlib/EtherCAT PDO Receive  Priority=2  sig_name=Box 1 (Degital Servo Adapter).HS-IN-AX03.AX03-HSI02  sig_offset=856  sig_type=int16  type_size=16  sig_dim=1  device_id=0  sample_time=0.000250
  FromDSA J4TrqCmd3 : xpcethercatlib/EtherCAT PDO Receive  Priority=2  sig_name=Box 1 (Degital Servo Adapter).HS-IN-AX04.AX04-HSI02  sig_offset=1112  sig_type=int16  type_size=16  sig_dim=1  device_id=0  sample_time=0.000250
  FromDSA J5TrqCmd4 : xpcethercatlib/EtherCAT PDO Receive  Priority=2  sig_name=Box 2 (Degital Servo Adapter).HS-IN-AX01.AX01-HSI02  sig_offset=2648  sig_type=int16  type_size=16  sig_dim=1  device_id=0  sample_time=0.000250
  FromDSA J6TrqCmd5 : xpcethercatlib/EtherCAT PDO Receive  Priority=2  sig_name=Box 2 (Degital Servo Adapter).HS-IN-AX02.AX02-HSI02  sig_offset=2904  sig_type=int16  type_size=16  sig_dim=1  device_id=0  sample_time=0.000250
  Mux : Mux  Inputs=6
  Rate Transition : RateTransition  OutPortSampleTime=si.tsv
  TrqCmdOut : Outport
  wires:
  FromDSA J6TrqCmd5/1 -> Mux/6
  FromDSA J4TrqCmd3/1 -> Mux/4
  FromDSA J2TrqCmd/1 -> Mux/2
  FromDSA J5TrqCmd4/1 -> Mux/5
  FromDSA J3TrqCmd2/1 -> Mux/3
  FromDSA J1TrqCmd/1 -> Mux/1
  Mux/1 -> Rate Transition/1
  Rate Transition/1 -> TrqCmdOut/1

== system LRMate200Experimentor_RobotState/Not Used/DSA System Variant/DSA System (Robot 1)/EtherCAT DSA TrqLimit ==
  In1 : Inport
  Conversion7 : DataTypeConversion
  Demux : Demux  Outputs=6
  "ToDSA J1TrqLimit " : xpcethercatlib/EtherCAT PDO Transmit   Priority=3  sig_name=Box 1 (Degital Servo Adapter).HS-OUT-AX01.AX01-HSO05  sig_offset=392  sig_type=int16  type_size=16  sig_dim=1  device_id=0  sample_time=0.000250
  ToDSA J2TrqLimit : xpcethercatlib/EtherCAT PDO Transmit   Priority=3  sig_name=Box 1 (Degital Servo Adapter).HS-OUT-AX02.AX02-HSO05  sig_offset=648  sig_type=int16  type_size=16  sig_dim=1  device_id=0  sample_time=0.000250
  ToDSA J3TrqLimit : xpcethercatlib/EtherCAT PDO Transmit   Priority=3  sig_name=Box 1 (Degital Servo Adapter).HS-OUT-AX03.AX03-HSO05  sig_offset=904  sig_type=int16  type_size=16  sig_dim=1  device_id=0  sample_time=0.000250
  ToDSA J4TrqLimit : xpcethercatlib/EtherCAT PDO Transmit   Priority=3  sig_name=Box 1 (Degital Servo Adapter).HS-OUT-AX04.AX04-HSO05  sig_offset=1160  sig_type=int16  type_size=16  sig_dim=1  device_id=0  sample_time=0.000250
  ToDSA J5TrqLimit : xpcethercatlib/EtherCAT PDO Transmit   Priority=3  sig_name=Box 2 (Degital Servo Adapter).HS-OUT-AX01.AX01-HSO05  sig_offset=2696  sig_type=int16  type_size=16  sig_dim=1  device_id=0  sample_time=0.000250
  ToDSA J6TrqLimit : xpcethercatlib/EtherCAT PDO Transmit   Priority=3  sig_name=Box 2 (Degital Servo Adapter).HS-OUT-AX02.AX02-HSO05  sig_offset=2952  sig_type=int16  type_size=16  sig_dim=1  device_id=0  sample_time=0.000250
  wires:
  In1/1 -> Conversion7/1
  Demux/1 -> "ToDSA J1TrqLimit "/1
  Demux/2 -> ToDSA J2TrqLimit/1
  Demux/3 -> ToDSA J3TrqLimit/1
  Demux/4 -> ToDSA J4TrqLimit/1
  Demux/5 -> ToDSA J5TrqLimit/1
  Demux/6 -> ToDSA J6TrqLimit/1
  Conversion7/1 -> Demux/1

== system LRMate200Experimentor_RobotState/Not Used/DSA System Variant/DSA System (Robot 1)/EtherCAT DSA VelOut ==
  FromDSA J1Vel : xpcethercatlib/EtherCAT PDO Receive  Priority=2  sig_name=Box 1 (Degital Servo Adapter).HS-IN-AX01.AX01-HSI10  sig_offset=472  sig_type=int32  type_size=32  sig_dim=1  device_id=0  sample_time=0.000250
  FromDSA J2Vel : xpcethercatlib/EtherCAT PDO Receive  Priority=2  sig_name=Box 1 (Degital Servo Adapter).HS-IN-AX02.AX02-HSI10  sig_offset=728  sig_type=int32  type_size=32  sig_dim=1  device_id=0  sample_time=0.000250
  FromDSA J3Vel : xpcethercatlib/EtherCAT PDO Receive  Priority=2  sig_name=Box 1 (Degital Servo Adapter).HS-IN-AX03.AX03-HSI10  sig_offset=984  sig_type=int32  type_size=32  sig_dim=1  device_id=0  sample_time=0.000250
  FromDSA J4Vel : xpcethercatlib/EtherCAT PDO Receive  Priority=2  sig_name=Box 1 (Degital Servo Adapter).HS-IN-AX04.AX04-HSI10  sig_offset=1240  sig_type=int32  type_size=32  sig_dim=1  device_id=0  sample_time=0.000250
  FromDSA J5Vel : xpcethercatlib/EtherCAT PDO Receive  Priority=2  sig_name=Box 2 (Degital Servo Adapter).HS-IN-AX01.AX01-HSI10  sig_offset=2776  sig_type=int32  type_size=32  sig_dim=1  device_id=0  sample_time=0.000250
  FromDSA J6Vel : xpcethercatlib/EtherCAT PDO Receive  Priority=2  sig_name=Box 2 (Degital Servo Adapter).HS-IN-AX02.AX02-HSI10  sig_offset=3032  sig_type=int32  type_size=32  sig_dim=1  device_id=0  sample_time=0.000250
  Mux : Mux  Inputs=6
  Rate Transition : RateTransition  OutPortSampleTime=si.tsv
  VelOut : Outport
  wires:
  FromDSA J6Vel/1 -> Mux/6
  FromDSA J4Vel/1 -> Mux/4
  FromDSA J2Vel/1 -> Mux/2
  FromDSA J5Vel/1 -> Mux/5
  FromDSA J3Vel/1 -> Mux/3
  FromDSA J1Vel/1 -> Mux/1
  Rate Transition/1 -> VelOut/1
  Mux/1 -> Rate Transition/1

== system LRMate200Experimentor_RobotState/Not Used/DSA System Variant/DSA System (Robot 2)/EtherCAT DSA AxEtcInfo ==
  FromDSA J1AxEtcInfo : xpcethercatlib/EtherCAT PDO Receive  Priority=2  sig_name=Box 3 (Degital Servo Adapter).NS-IN-AX01.AX01-NSI07  sig_offset=6312  sig_type=uint16  type_size=16  sig_dim=1  device_id=0  sample_time=0.000250
  FromDSA J2AxEtcInfo : xpcethercatlib/EtherCAT PDO Receive  Priority=2  sig_name=Box 3 (Degital Servo Adapter).NS-IN-AX02.AX02-NSI07  sig_offset=6504  sig_type=uint16  type_size=16  sig_dim=1  device_id=0  sample_time=0.000250
  FromDSA J3AxEtcInfo : xpcethercatlib/EtherCAT PDO Receive  Priority=2  sig_name=Box 3 (Degital Servo Adapter).NS-IN-AX03.AX03-NSI07  sig_offset=6696  sig_type=uint16  type_size=16  sig_dim=1  device_id=0  sample_time=0.000250
  FromDSA J4AxEtcInfo : xpcethercatlib/EtherCAT PDO Receive  Priority=2  sig_name=Box 3 (Degital Servo Adapter).NS-IN-AX04.AX04-NSI07  sig_offset=6888  sig_type=uint16  type_size=16  sig_dim=1  device_id=0  sample_time=0.000250
  FromDSA J5AxEtcInfo : xpcethercatlib/EtherCAT PDO Receive  Priority=2  sig_name=Box 4 (Degital Servo Adapter).NS-IN-AX01.AX01-NSI07  sig_offset=8616  sig_type=uint16  type_size=16  sig_dim=1  device_id=0  sample_time=0.000250
  FromDSA J6AxEtcInfo : xpcethercatlib/EtherCAT PDO Receive  Priority=2  sig_name=Box 4 (Degital Servo Adapter).NS-IN-AX02.AX02-NSI07  sig_offset=8808  sig_type=uint16  type_size=16  sig_dim=1  device_id=0  sample_time=0.000250
  Mux : Mux  Inputs=6
  Rate Transition : RateTransition  OutPortSampleTime=si.tsv
  AxEtcInfoOut : Outport
  wires:
  FromDSA J6AxEtcInfo/1 -> Mux/6
  FromDSA J4AxEtcInfo/1 -> Mux/4
  FromDSA J2AxEtcInfo/1 -> Mux/2
  FromDSA J5AxEtcInfo/1 -> Mux/5
  FromDSA J3AxEtcInfo/1 -> Mux/3
  FromDSA J1AxEtcInfo/1 -> Mux/1
  Mux/1 -> Rate Transition/1
  Rate Transition/1 -> AxEtcInfoOut/1
